simulink model "simulink_first_order"  (R2020b)
settings: Solver=VariableStepAuto  StartTime=0.0  StopTime=0.1  RelTol=1e-3
settings Model: Creator=99003757  LastModifiedBy=99003727

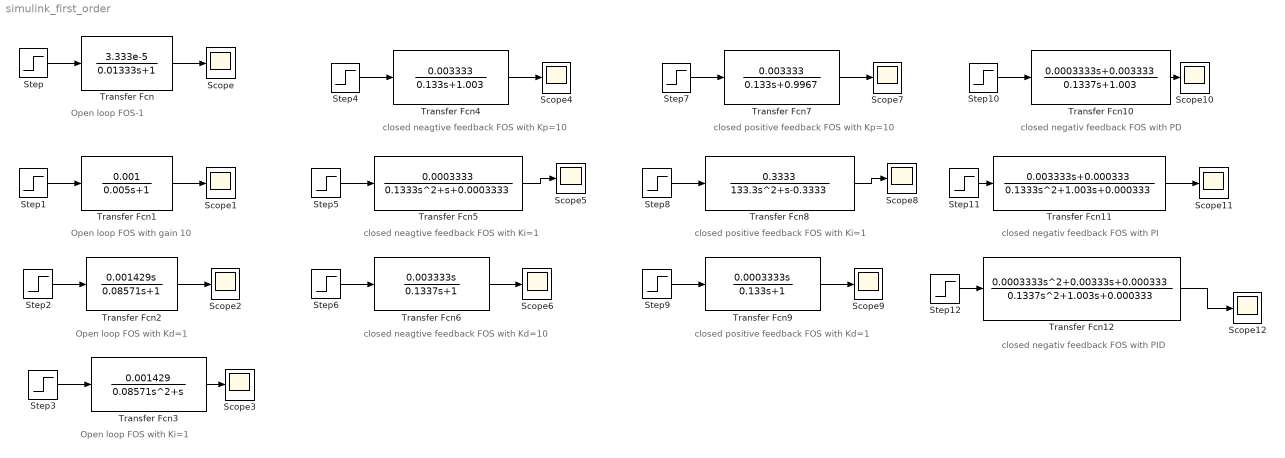
== system simulink_first_order ==
  note: Open loop FOS-1
  note: Open loop FOS with gain 10
  note: Open loop FOS with Kd=1
  note: Open loop FOS with Ki=1
  note: closed neagtive feedback FOS with Kp=10
  note: closed neagtive feedback FOS with Ki=1
  note: closed neagtive feedback FOS with Kd=10
  note: closed positive feedback FOS with Kp=10
  note: closed positive feedback FOS with Ki=1
  note: closed positive feedback FOS with Kd=1
  note: closed negativ feedback FOS with PID
  note: closed negativ feedback FOS with PD
  note: closed negativ feedback FOS with PI
  Scope{,1..12} (13 alike) : Scope
  Step{,1..12} (13 alike) : Step  Time=0  SampleTime=0
  Transfer Fcn : TransferFcn  Numerator=[3.333e-5]  Denominator=[0.01333 1]
  Transfer Fcn1 : TransferFcn  Numerator=[0.001]  Denominator=[0.005 1]
  Transfer Fcn10 : TransferFcn  Numerator=[0.0003333 0.003333 ]  Denominator=[0.1337 1.003]
  Transfer Fcn11 : TransferFcn  Numerator=[0.003333 0.000333 ]  Denominator=[0.1333 1.003 0.000333]
  Transfer Fcn12 : TransferFcn  Numerator=[0.0003333 0.00333 0.000333 ]  Denominator=[0.1337 1.003 0.000333]
  Transfer Fcn2 : TransferFcn  Numerator=[0.001429 0]  Denominator=[0.08571 1]
  Transfer Fcn3 : TransferFcn  Numerator=[0.001429]  Denominator=[0.08571 1 0]
  Transfer Fcn4 : TransferFcn  Numerator=[0.003333]  Denominator=[0.133 1.003]
  Transfer Fcn5 : TransferFcn  Numerator=[0.0003333]  Denominator=[0.1333 1 0.0003333]
  Transfer Fcn6 : TransferFcn  Numerator=[0.003333 0]  Denominator=[0.1337 1]
  Transfer Fcn7 : TransferFcn  Numerator=[0.003333]  Denominator=[0.133 0.9967]
  Transfer Fcn8 : TransferFcn  Numerator=[0.3333]  Denominator=[133.3 1 -0.3333]
  Transfer Fcn9 : TransferFcn  Numerator=[0.0003333 0]  Denominator=[0.133 1]
  wires:
  Transfer Fcn/1 -> Scope/1
  Step/1 -> Transfer Fcn/1
  Transfer Fcn1/1 -> Scope1/1
  Step1/1 -> Transfer Fcn1/1
  Step2/1 -> Transfer Fcn2/1
  Transfer Fcn2/1 -> Scope2/1
  Step3/1 -> Transfer Fcn3/1
  Transfer Fcn3/1 -> Scope3/1
  Step4/1 -> Transfer Fcn4/1
  Transfer Fcn4/1 -> Scope4/1
  Transfer Fcn5/1 -> Scope5/1
  Step5/1 -> Transfer Fcn5/1
  Transfer Fcn6/1 -> Scope6/1
  Step6/1 -> Transfer Fcn6/1
  Transfer Fcn7/1 -> Scope7/1
  Step7/1 -> Transfer Fcn7/1
  Step8/1 -> Transfer Fcn8/1
  Transfer Fcn8/1 -> Scope8/1
  Transfer Fcn9/1 -> Scope9/1
  Step9/1 -> Transfer Fcn9/1
  Step12/1 -> Transfer Fcn12/1
  Transfer Fcn11/1 -> Scope11/1
  Step10/1 -> Transfer Fcn10/1
  Transfer Fcn12/1 -> Scope12/1
  Step11/1 -> Transfer Fcn11/1
  Transfer Fcn10/1 -> Scope10/1
